simulink model "HFI_Simulation"  (R2023a)
settings: Solver=VariableStepAuto  StartTime=0.0  StopTime=10.0  RelTol=1e-3
libraries: simulink x1
settings Model: Creator=洲  LastModifiedBy=洲

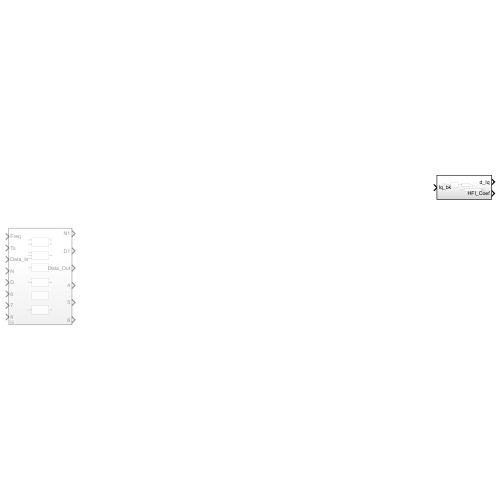
[thumbnail: Simulink's stored preview of the top-level diagram]
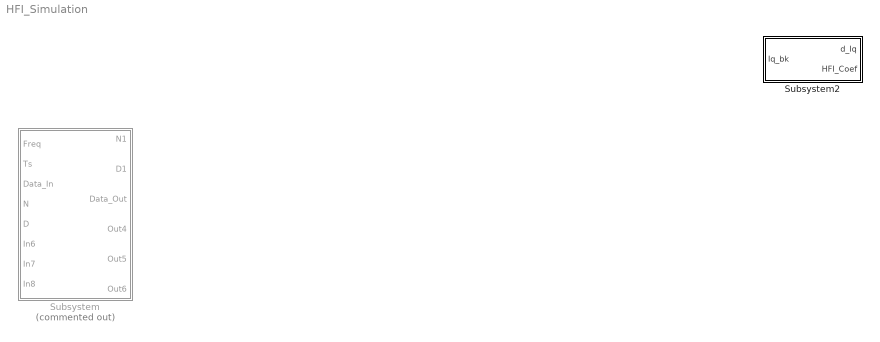
== system HFI_Simulation ==
  Subsystem : Subsystem  Commented=on
  Subsystem2 : Subsystem

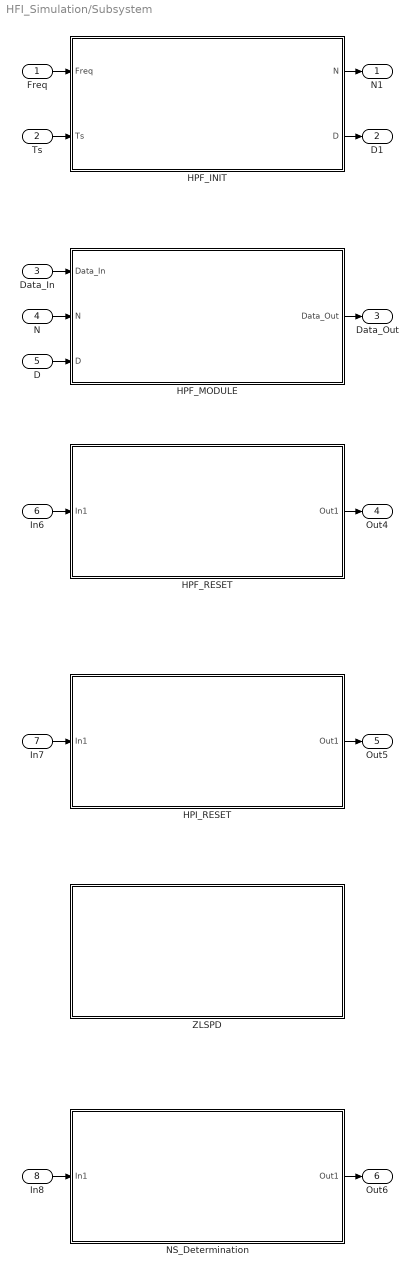
== system HFI_Simulation/Subsystem ==
  Freq : Inport
  Ts : Inport  Port=2
  Data_In : Inport  Port=3
  N : Inport  Port=4
  D : Inport  Port=5
  In6 : Inport  Port=6
  In7 : Inport  Port=7
  In8 : Inport  Port=8
  HPF_INIT : Subsystem
  HPF_MODULE : Subsystem
  HPF_RESET : Subsystem
  HPI_RESET : Subsystem
  NS_Determination : Subsystem
  ZLSPD : Subsystem
  N1 : Outport
  D1 : Outport  Port=2
  Data_Out : Outport  Port=3
  Out4 : Outport  Port=4
  Out5 : Outport  Port=5
  Out6 : Outport  Port=6
  wires:
  HPF_RESET/1(Out1) -> Out4/1
  HPF_INIT/1(N) -> N1/1
  Ts/1 -> HPF_INIT/2(Ts)
  N/1 -> HPF_MODULE/2(N)
  HPI_RESET/1(Out1) -> Out5/1
  In7/1 -> HPI_RESET/1(In1)
  Freq/1 -> HPF_INIT/1(Freq)
  HPF_MODULE/1(Data_Out) -> Data_Out/1
  HPF_INIT/2(D) -> D1/1
  In8/1 -> NS_Determination/1(In1)
  NS_Determination/1(Out1) -> Out6/1
  Data_In/1 -> HPF_MODULE/1(Data_In)
  In6/1 -> HPF_RESET/1(In1)
  D/1 -> HPF_MODULE/3(D)

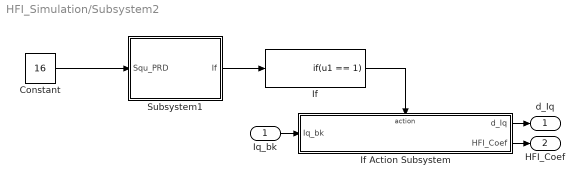
== system HFI_Simulation/Subsystem2 ==
  Iq_bk : Inport
  Constant : Constant  Value=16  OutDataTypeStr=uint8
  If : If  IfExpression=u1 == 1  ShowElse=off
  If Action Subsystem : Subsystem  TreatAsAtomicUnit=on
  Subsystem1 : Subsystem
  d_Iq : Outport
  HFI_Coef : Outport  Port=2
  wires:
  Subsystem1/1(If) -> If/1
  If/1 -> If Action Subsystem/Action
  If Action Subsystem/2(HFI_Coef) -> HFI_Coef/1
  Constant/1 -> Subsystem1/1(Squ_PRD)
  Iq_bk/1 -> If Action Subsystem/1(Iq_bk)
  If Action Subsystem/1(d_Iq) -> d_Iq/1

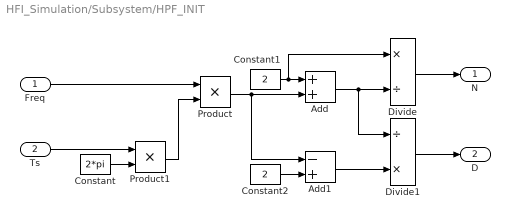
== system HFI_Simulation/Subsystem/HPF_INIT ==
  Freq : Inport
  Ts : Inport  Port=2
  Add : Sum
  Add1 : Sum  Inputs=-+
  Constant : Constant  Value=2*pi  OutDataTypeStr=single
  Constant1 : Constant  Value=2  OutDataTypeStr=single
  Constant2 : Constant  Value=2  OutDataTypeStr=single
  Divide : Product  Inputs=*/
  Divide1 : Product  Inputs=/*
  Product : Product
  Product1 : Product
  N : Outport
  D : Outport  Port=2
  wires:
  Freq/1 -> Product/1
  Ts/1 -> Product1/1
  Constant/1 -> Product1/2
  Product1/1 -> Product/2
  Product/1 -> Add1/1, Add/2
  Constant1/1 -> Divide/1, Add/1
  Add/1 -> Divide1/1, Divide/2
  Divide/1 -> N/1
  Constant2/1 -> Add1/2
  Add1/1 -> Divide1/2
  Divide1/1 -> D/1

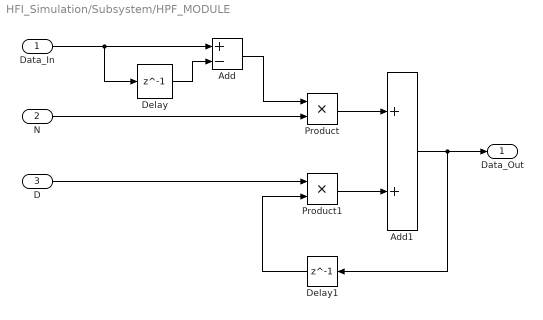
== system HFI_Simulation/Subsystem/HPF_MODULE ==
  Data_In : Inport
  N : Inport  Port=2
  D : Inport  Port=3
  Add : Sum  Inputs=+-
  Add1 : Sum
  Delay : Delay  DelayLength=1
  Delay1 : Delay  DelayLength=1
  Product : Product
  Product1 : Product
  Data_Out : Outport
  wires:
  Data_In/1 -> Add/1, Delay/1
  Delay/1 -> Add/2
  Add/1 -> Product/1
  N/1 -> Product/2
  D/1 -> Product1/1
  Delay1/1 -> Product1/2
  Product/1 -> Add1/1
  Add1/1 -> Delay1/1, Data_Out/1
  Product1/1 -> Add1/2

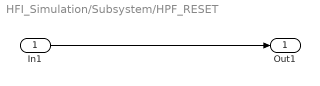
== system HFI_Simulation/Subsystem/HPF_RESET ==
  In1 : Inport
  Out1 : Outport
  wires:
  In1/1 -> Out1/1

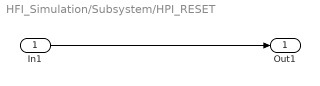
== system HFI_Simulation/Subsystem/HPI_RESET ==
  In1 : Inport
  Out1 : Outport
  wires:
  In1/1 -> Out1/1

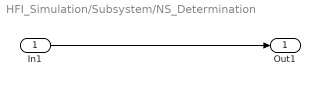
== system HFI_Simulation/Subsystem/NS_Determination ==
  In1 : Inport
  Out1 : Outport
  wires:
  In1/1 -> Out1/1

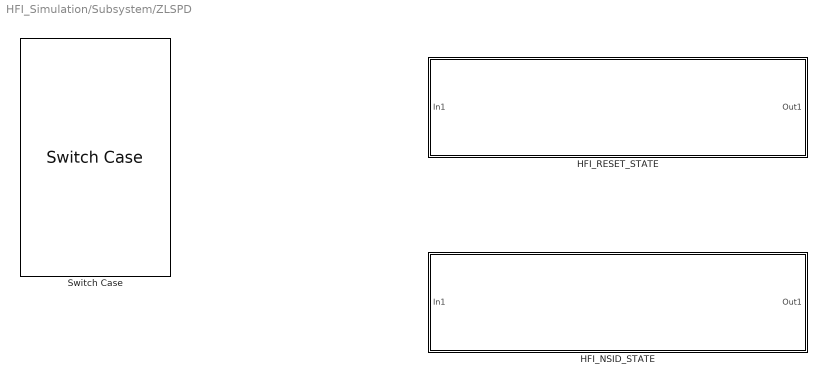
== system HFI_Simulation/Subsystem/ZLSPD ==
  HFI_NSID_STATE : Subsystem
  HFI_RESET_STATE : Subsystem
  Switch Case : SwitchCase  CaseConditions={0,1,2,3}

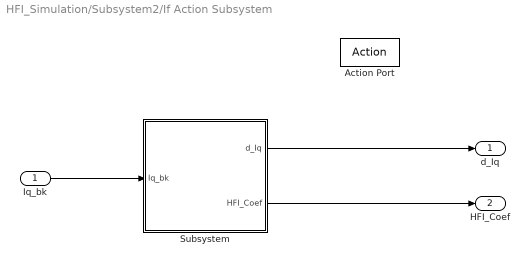
== system HFI_Simulation/Subsystem2/If Action Subsystem ==
  Iq_bk : Inport
  Action Port : ActionPort  ActionPortLabel=if(u1 == 1)
  Subsystem : Subsystem
  d_Iq : Outport
  HFI_Coef : Outport  Port=2
  wires:
  Iq_bk/1 -> Subsystem/1(Iq_bk)
  Subsystem/1(d_Iq) -> d_Iq/1
  Subsystem/2(HFI_Coef) -> HFI_Coef/1

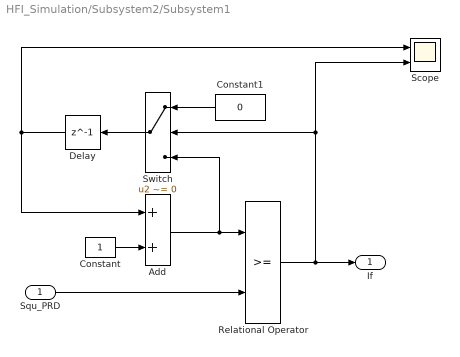
== system HFI_Simulation/Subsystem2/Subsystem1 ==
  Squ_PRD : Inport
  Add : Sum
  Constant : Constant  OutDataTypeStr=uint8
  Constant1 : Constant  Value=0  OutDataTypeStr=uint8
  Delay : Delay  DelayLength=1
  Relational Operator : RelationalOperator  OutDataTypeStr=boolean  RndMeth=Simplest  InputSameDT=off
  Scope : Scope  NumInputPorts=2
  Switch : Switch  Criteria=u2 ~= 0  SaturateOnIntegerOverflow=off  InputSameDT=off
  If : Outport
  wires:
  Delay/1 -> Scope/1, Add/1
  Constant/1 -> Add/2
  Squ_PRD/1 -> Relational Operator/2
  Relational Operator/1 -> If/1, Scope/2, Switch/2
  Add/1 -> Switch/3, Relational Operator/1
  Constant1/1 -> Switch/1
  Switch/1 -> Delay/1

== system HFI_Simulation/Subsystem/ZLSPD/HFI_NSID_STATE ==
  In1 : Inport
  Out1 : Outport
  wires:
  In1/1 -> Out1/1

== system HFI_Simulation/Subsystem/ZLSPD/HFI_RESET_STATE ==
  In1 : Inport
  Out1 : Outport
  wires:
  In1/1 -> Out1/1

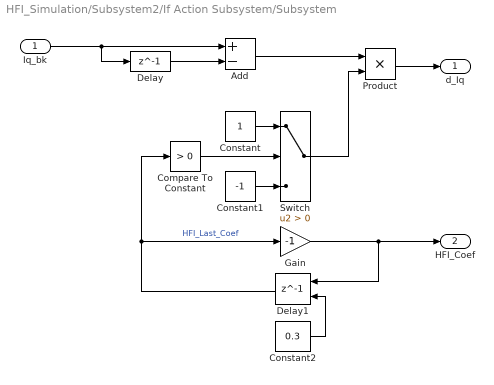
== system HFI_Simulation/Subsystem2/If Action Subsystem/Subsystem ==
  Iq_bk : Inport
  Add : Sum  Inputs=+-
  Compare To Constant : simulink/Logic and Bit Operations/Compare To Constant  relop=>  const=0  OutDataTypeStr=boolean
  Constant : Constant  OutDataTypeStr=single
  Constant1 : Constant  Value=-1  OutDataTypeStr=single
  Constant2 : Constant  Value=0.3
  Delay : Delay  DelayLength=1
  Delay1 : Delay  DelayLength=1  InitialConditionSource=Input port
      settings: InputPortMap=u0,p4
  Gain : Gain  Gain=-1
  Product : Product
  Switch : Switch  Criteria=u2 > Threshold  SaturateOnIntegerOverflow=off  InputSameDT=off
  d_Iq : Outport
  HFI_Coef : Outport  Port=2
  wires:
  Constant/1 -> Switch/1
  Constant1/1 -> Switch/3
  Delay1/1 -> Gain/1, Compare To Constant/1  "HFI_Last_Coef"
  Product/1 -> d_Iq/1
  Delay/1 -> Add/2
  Gain/1 -> HFI_Coef/1, Delay1/1
  Iq_bk/1 -> Delay/1, Add/1
  Compare To Constant/1 -> Switch/2
  Switch/1 -> Product/2
  Constant2/1 -> Delay1/2
  Add/1 -> Product/1
